simulink model "Laba5slx"  (R2018b)
settings: Solver=VariableStepAuto  StartTime=0.0  StopTime=10.0  RelTol=1e-3
undefined symbols (not defined in the file): bB
libraries: dspsnks4 x2, dspvision x2, dspsrcs4 x2
settings Model: Creator=Student  LastModifiedBy=Student

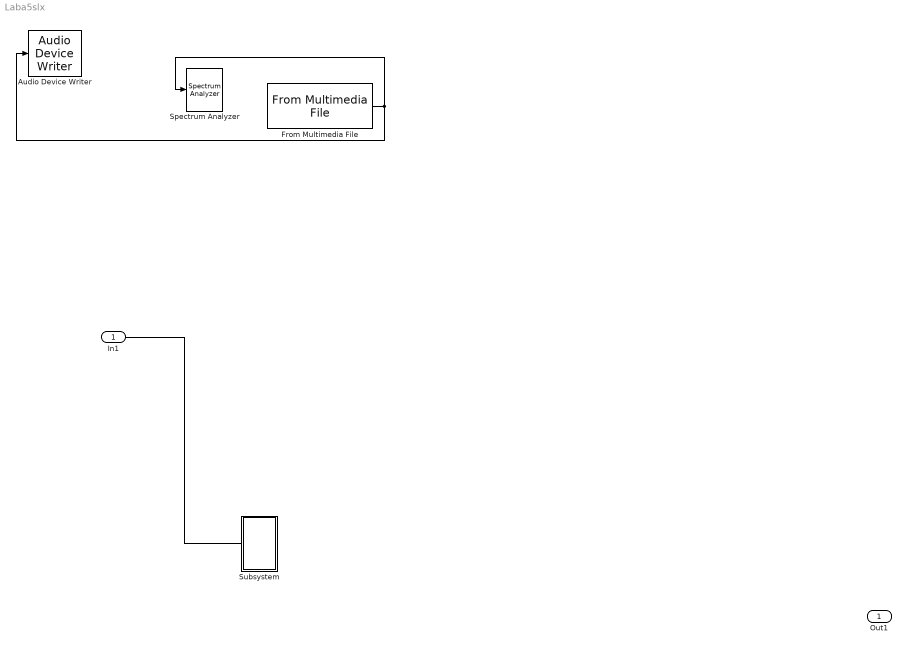
== system Laba5slx ==
  In1 : Inport
  Audio Device Writer : dspsnks4/Audio Device Writer  Driver=DirectSound  Device=Default  InheritSampleRate=on  SampleRate=44100  BitDepth=16-bit integer  BufferSize=4096  NumBuffers=10  DefaultOutputChannelMapping=on  OutputChannelMapping=1:2  OutputNumUnderrunSamples=off  DriverIdx=1  DeviceWarnFlag=''
  From Multimedia File : dspvision/From Multimedia File  inputFilename=Z:\2_course\4931101_10002\song.mp3  loop=on  numPlays=inf  outputStreams=Audio only  videoDataType=single  audioDataType=double  inheritSampleTime=on  userDefinedSampleTime=1/30  noAudioOutput=off  isIntensityVideo=off  fourcc=RGB  colorVideoFormat=Separate color signals  outputEOF=off  dataOrg=Column-major  audioFrameSize=1024  computeAudioFrameSize=off  outSamplingMode=Sample based
      settings: SourceProductBaseCode=VP
  Spectrum Analyzer : SpectrumAnalyzer
  Subsystem : Subsystem
  Out1 : Outport
  wires:
  From Multimedia File/1 -> Spectrum Analyzer/1, Audio Device Writer/1
  In1/1 -> ?
  ? -> Out1/1

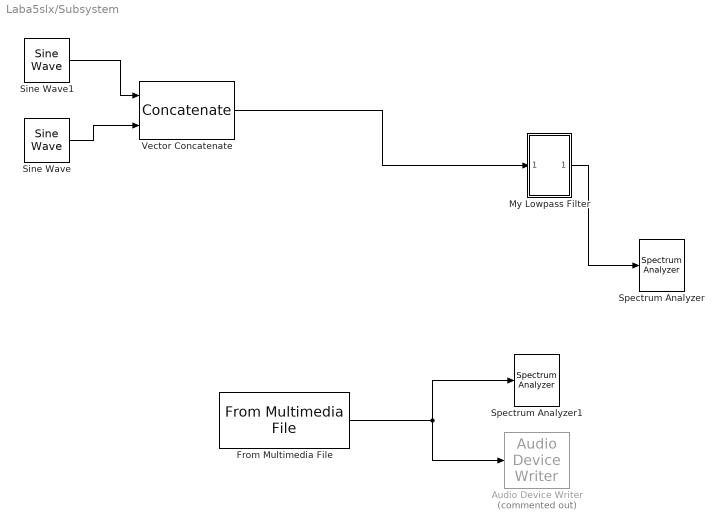
== system Laba5slx/Subsystem ==
  Audio Device Writer : dspsnks4/Audio Device Writer  Commented=on  Driver=DirectSound  Device=Default  InheritSampleRate=on  SampleRate=44100  BitDepth=16-bit integer  BufferSize=4096  NumBuffers=10  DefaultOutputChannelMapping=on  OutputChannelMapping=1:2  OutputNumUnderrunSamples=off  DriverIdx=1  DeviceWarnFlag=''
  From Multimedia File : dspvision/From Multimedia File  inputFilename=Z:\2_course\4931101_10002\song.mp3  loop=on  numPlays=inf  outputStreams=Audio only  videoDataType=single  audioDataType=double  inheritSampleTime=on  userDefinedSampleTime=1/30  noAudioOutput=off  isIntensityVideo=off  fourcc=RGB  colorVideoFormat=Separate color signals  outputEOF=off  dataOrg=Column-major  audioFrameSize=1024  computeAudioFrameSize=off  outSamplingMode=Sample based
      settings: SourceProductBaseCode=VP
  My Lowpass Filter : Subsystem
  Sine Wave : dspsrcs4/Sine Wave  Amplitude=1  Frequency=17000  Phase=0  SampleMode=Discrete  OutComplex=Real  CompMethod=Trigonometric fcn  TableSize=Speed  SampleTime=1/44100  SamplesPerFrame=1024  ResetState=Restart at time zero  OutputFrames=off  dataType=double  wordLen=16  udDataType=sfix(16)  fracBitsMode=Best precision  numFracBits=15  OutDataTypeStr=double  LastOutDataTypeStr=double
  Sine Wave1 : dspsrcs4/Sine Wave  Amplitude=1  Frequency=17000  Phase=0  SampleMode=Discrete  OutComplex=Real  CompMethod=Trigonometric fcn  TableSize=Speed  SampleTime=1/44100  SamplesPerFrame=1024  ResetState=Restart at time zero  OutputFrames=off  dataType=double  wordLen=16  udDataType=sfix(16)  fracBitsMode=Best precision  numFracBits=15  OutDataTypeStr=double  LastOutDataTypeStr=double
  Spectrum Analyzer : SpectrumAnalyzer
  Spectrum Analyzer1 : SpectrumAnalyzer
  Vector Concatenate : Concatenate  Mode=Multidimensional array  ConcatenateDimension=2
  wires:
  Sine Wave1/1 -> Vector Concatenate/1
  Sine Wave/1 -> Vector Concatenate/2
  My Lowpass Filter/1(Out1) -> Spectrum Analyzer/1
  Vector Concatenate/1 -> My Lowpass Filter/1(In1)
  From Multimedia File/1 -> Audio Device Writer/1, Spectrum Analyzer1/1

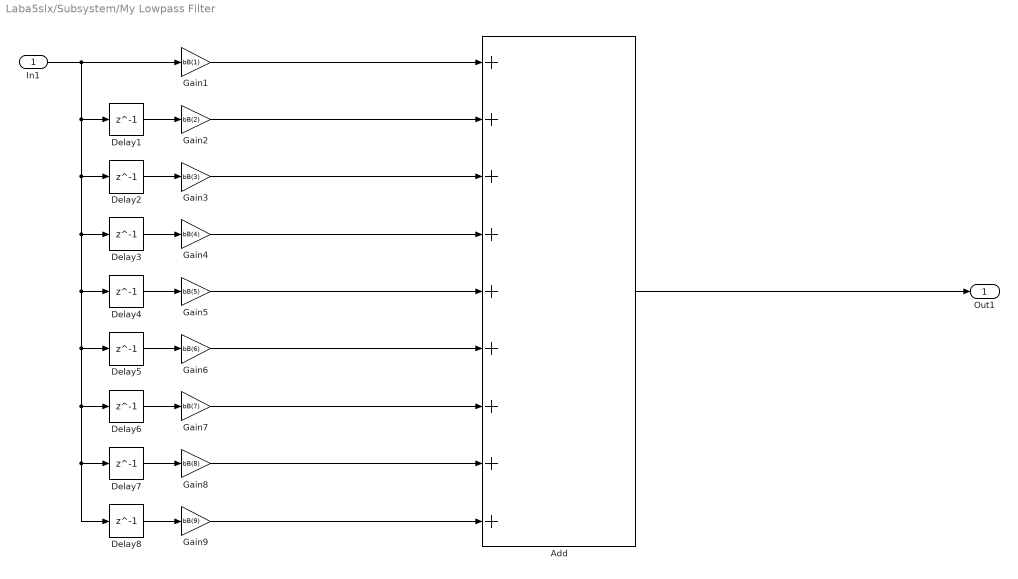
== system Laba5slx/Subsystem/My Lowpass Filter ==
  In1 : Inport
  Add : Sum  Inputs=+++++++++
  Delay{1..8} (8 alike) : Delay  DelayLength=1  InitialCondition=0
  Gain1 : Gain  Gain=bB(1)
  Gain2 : Gain  Gain=bB(2)
  Gain3 : Gain  Gain=bB(3)
  Gain4 : Gain  Gain=bB(4)
  Gain5 : Gain  Gain=bB(5)
  Gain6 : Gain  Gain=bB(6)
  Gain7 : Gain  Gain=bB(7)
  Gain8 : Gain  Gain=bB(8)
  Gain9 : Gain  Gain=bB(9)
  Out1 : Outport
  wires:
  Gain1/1 -> Add/1
  Delay8/1 -> Gain9/1
  Gain6/1 -> Add/6
  Gain7/1 -> Add/7
  Gain2/1 -> Add/2
  Delay4/1 -> Gain5/1
  Gain9/1 -> Add/9
  Gain8/1 -> Add/8
  Gain5/1 -> Add/5
  In1/1 -> Gain1/1, Delay1/1, Delay5/1, Delay6/1, Delay7/1, Delay8/1, Delay4/1, Delay3/1, Delay2/1
  Gain3/1 -> Add/3
  Gain4/1 -> Add/4
  Delay3/1 -> Gain4/1
  Delay6/1 -> Gain7/1
  Add/1 -> Out1/1
  Delay5/1 -> Gain6/1
  Delay7/1 -> Gain8/1
  Delay1/1 -> Gain2/1
  Delay2/1 -> Gain3/1
